simulink model "IMUSim"  (Simulink 7.7)
settings: Solver=FixedStepDiscrete  StartTime=0.0  StopTime=T_Stop  FixedStep=T  MaxStep=0.0058072  RelTol=1e-3
settings Model: Creator=kutenai  LastModifiedBy=kutenai
settings OptimizationCC: BooleanDataType=off  InlineInvariantSignals=on  InitFltsAndDblsToZero=on
settings DebuggingCC: SaveWithParameterizedLinksMsg=none  SignalResolutionControl=TryResolveAllWithWarning  SolverPrmCheckMsg=none  MultiTaskDSMMsg=warning  MultiTaskCondExecSysMsg=none  StrictBusMsg=None
settings HardwareCC: TargetUnknown=on
settings RTWCC: IncludeERTFirstTime=on
settings GRTTargetCC: TargetFcnLib=ansi_tfl_tmw.mat  ModelReferenceCompliant=off  ParMdlRefBuildCompliant=off  CompOptLevelCompliant=off  MatFileLogging=off

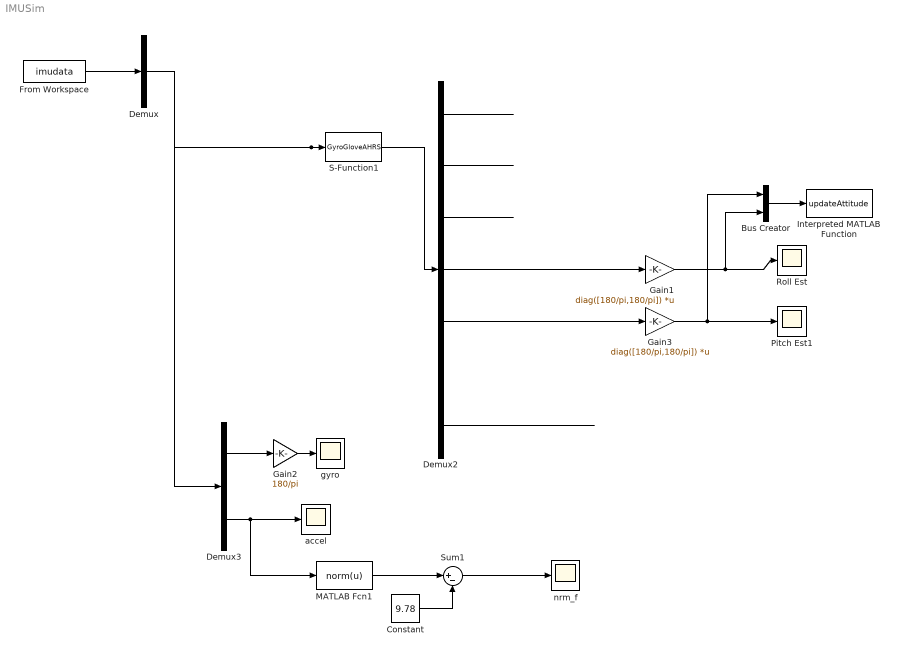
== system IMUSim ==
  Bus Creator : BusCreator  Inputs=2
  Constant : Constant  Value=9.78
  Demux : Demux  Outputs=1
  Demux2 : Demux  Outputs=[4,3,3,2,2,2,2]
  Demux3 : Demux  Outputs=[3,3]
  From Workspace : FromWorkspace  VariableName=imudata  SampleTime=1/180
  Gain1 : Gain  Gain=diag([180/pi,180/pi])  Multiplication=Matrix(K*u)  SaturateOnIntegerOverflow=on  OutDataTypeStr=Inherit: Same as input  ParamDataTypeStr=Inherit: Same as input
  Gain2 : Gain  Gain=180/pi  SaturateOnIntegerOverflow=on  OutDataTypeStr=Inherit: Same as input  ParamDataTypeStr=Inherit: Same as input
  Gain3 : Gain  Gain=diag([180/pi,180/pi])  Multiplication=Matrix(K*u)  SaturateOnIntegerOverflow=on  OutDataTypeStr=Inherit: Same as input  ParamDataTypeStr=Inherit: Same as input
  Interpreted MATLAB Function : MATLABFcn  MATLABFcn=updateAttitude
  MATLAB Fcn1 : MATLABFcn  MATLABFcn=norm(u)
  Pitch Est1 : Scope
      settings: TimeRange=10  YMin=-100  YMax=100
  Roll Est : Scope
      settings: TimeRange=10  YMin=-200  YMax=200  SaveName=ScopeData3
  S-Function1 : S-Function  FunctionName=GyroGloveAHRS  EnableBusSupport=off
  Sum1 : Sum  Inputs=|+-  SaturateOnIntegerOverflow=on  InputSameDT=on  OutDataTypeStr=Inherit: Same as first input
  accel : Scope
      settings: TimeRange=300  YMin=-20  YMax=20  SaveName=ScopeData8
  gyro : Scope
      settings: TimeRange=300  YMin=-100  YMax=100  SaveName=ScopeData6
  nrm_f : Scope
      settings: TimeRange=300  YMin=-1  YMax=1  SaveName=ScopeData15
  wires:
  Demux/1 -> S-Function1/1, Demux3/1
  S-Function1/1 -> Demux2/1
  Demux2/4 -> Gain1/1
  Demux3/1 -> Gain2/1
  Demux3/2 -> accel/1, MATLAB Fcn1/1
  Demux2/2 -> ?
  Demux2/3 -> ?
  Gain1/1 -> Roll Est/1, Bus Creator/2
  Demux2/1 -> ?
  MATLAB Fcn1/1 -> Sum1/1
  Sum1/1 -> nrm_f/1
  Constant/1 -> Sum1/2
  From Workspace/1 -> Demux/1
  Gain2/1 -> gyro/1
  Demux2/7 -> ?
  Gain3/1 -> Pitch Est1/1, Bus Creator/1
  Demux2/5 -> Gain3/1
  Bus Creator/1 -> Interpreted MATLAB Function/1
